simulink model "example"  (Simulink 8.5)
settings: Solver=ode4  StartTime=0.0  StopTime=inf  FixedStep=0.01  RelTol=1e-3
libraries: MAVLink2Simulink_Serial x1, aerolibanimutils x1
settings Model: Creator=ttcl3  LastModifiedBy=David
settings DebuggingCC: SolverPrmCheckMsg=warning  FcnCallInpInsideContextMsg=UseLocalSettings

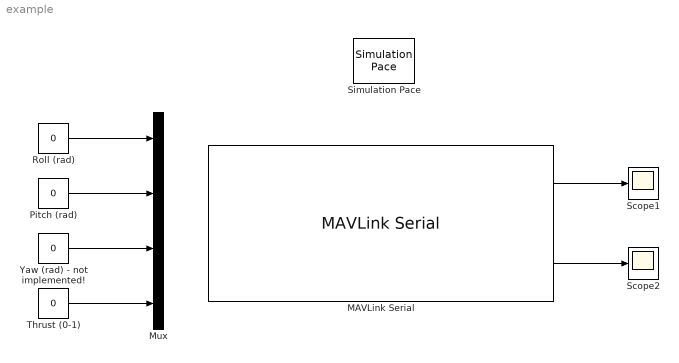
== system example ==
  MAVLink Serial : MAVLink2Simulink_Serial/MAVLink Serial  COM_Port='COM4'  Baud_Rate=115200  HEART_BEAT=off  ATTITUDE_OUT=on  RAW_IMU=on  POSITION_OUT=off  VFR_HUD=off  RC_SCALED=off  SERVO_OUT_RAW=off  SET_MODE=off  DATA_STREAM=off  ATTITUDE_COMMAND=off  ATTITUDE_IN=off  GPS_RAW_IN=off  VFR_HUD_IN=off
  Mux : Mux
  Pitch (rad) : Constant  Value=0
  Roll (rad) : Constant  Value=0
  Scope1 : Scope
      settings: YMin=-0.1  YMax=0.1
  Scope2 : Scope
      settings: YMin=-0.85  YMax=0.15
  Simulation Pace : aerolibanimutils/Simulation Pace  SimulationPace=1  SleepMode=MATLAB Thread  OutputPaceError=off  SampleTime=0.01
      settings: AttributesFormatString=%<SimulationPace> sec/sec
  Thrust (0-1) : Constant  Value=0
  Yaw (rad) - not implemented! : Constant  Value=0
  wires:
  Roll (rad)/1 -> Mux/1
  Pitch (rad)/1 -> Mux/2
  Yaw (rad) - not implemented!/1 -> Mux/3
  Thrust (0-1)/1 -> Mux/4
  MAVLink Serial/1 -> Scope1/1
  MAVLink Serial/2 -> Scope2/1
